simulink model "task8_simulink"  (R2024b)
settings: Solver=VariableStepAuto  StartTime=0.0  StopTime=100  RelTol=1e-3
values from neighbouring files (symbols this model uses):
  A = [ ... (first row only)    [longitudinal_linear_model.m]
  B = [ ... (first row only)    [longitudinal_linear_model.m]
  delta_trim = trim_solution(3)    [main.m]
  T_trim = trim_solution(1)    [main.m]
settings Model: Creator=Admin  LastModifiedBy=Admin

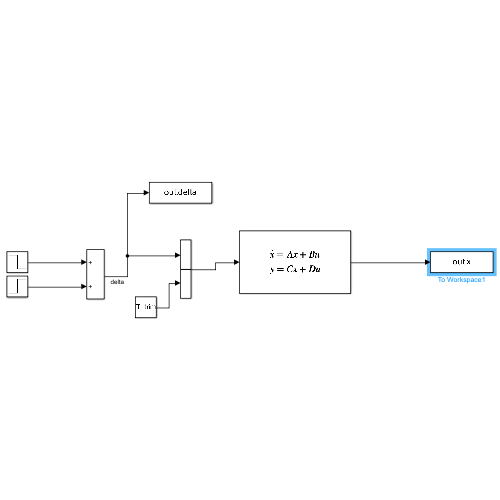
[thumbnail: Simulink's stored preview of the top-level diagram]
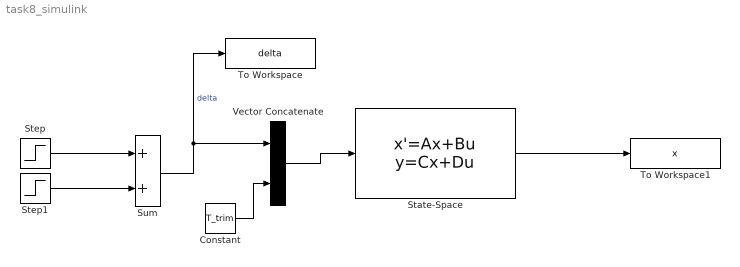
== system task8_simulink ==
  Constant : Constant  Value=T_trim
  State-Space : StateSpace  A=A  B=B  C=eye(4)  D=zeros(4,2)  InitialCondition=zeros(4,1)
  Step : Step  Time=5  Before=delta_trim  After=delta_trim - pi/180  SampleTime=0
  Step1 : Step  Time=10  After=(pi/180)  SampleTime=0
  Sum : Sum
  To Workspace : ToWorkspace  VariableName=delta  SampleTime=-1
  To Workspace1 : ToWorkspace  VariableName=x  SaveFormat=Structure  SampleTime=-1
      settings: Save2DSignal=2-D array (concatenate along first dimension)
  Vector Concatenate : Concatenate
  wires:
  Step/1 -> Sum/1
  Step1/1 -> Sum/2
  Sum/1 -> Vector Concatenate/1, To Workspace/1  "delta"
  State-Space/1 -> To Workspace1/1
  Vector Concatenate/1 -> State-Space/1
  Constant/1 -> Vector Concatenate/2
